simulink model "model_affc"  (R2016b)
settings: Solver=FixedStepDiscrete  StartTime=0.0  StopTime=inf  FixedStep=sampleTime  RelTol=1e-3
InitFcn:
  | model_affc_parameters;
StartFcn:
  | model_affc_parameters;
values from neighbouring files (symbols this model uses):
  Lb = 0.07    [model_affc_parameters.m]    (also in parameters_sysid.m)
  Lf = 0.238    [model_affc_parameters.m]    (also in parameters_sysid.m)
  Lu = 0.153    [model_affc_parameters.m]    (also in parameters_sysid.m)
  sampleTime = 0.001    [model_affc_parameters.m]    (also in parameters_sysid.m)
undefined symbols (not defined in the file or in its folder): FM1
libraries: simulink x4, LibraryFM x4, VariousBlocksLibrary x2, FMLibrary_v2 x1
settings Model: SimulationMode=external  Creator=niekbeckers  LastModifiedBy=Labuser
settings DataIOCC: LimitDataPoints=on  SaveFormat=Array
settings OptimizationCC: BlockReduction=off  BooleanDataType=off  LocalBlockOutputs=off  LifeSpan=inf
settings DebuggingCC: SaveWithParameterizedLinksMsg=none  UnderspecifiedInitializationDetection=Classic  MergeDetectMultiDrivingBlocksExec=none  SignalResolutionControl=TryResolveAllWithWarning  SFUnexpectedBacktrackingDiag=warning  SFNoUnconditionalDefaultTransitionDiag=warning  SFExecutionAtInitializationDiag=none
settings HardwareCC: ProdBitPerPointer=32  ProdBitPerSizeT=32  ProdBitPerPtrDiffT=32  ProdLargestAtomicFloat=None  ProdIntDivRoundTo=Undefined  ProdEndianess=Unspecified  ProdWordSize=32  ProdHWDeviceType=32-bit Generic  TargetBitPerPointer=64  TargetBitPerSizeT=64  TargetBitPerPtrDiffT=64  TargetLongLongMode=on  TargetIntDivRoundTo=Zero  TargetEndianess=LittleEndian  TargetWordSize=64  TargetHWDeviceType=MATLAB Host  ProdEqTarget=off
settings ModelReferenceCC: PropagateSignalLabelsOutOfModel=off
settings RTWCC: SystemTargetFile=TwinCAT.tlc  GenCodeOnly=on  MakeCommand=make_tct  TemplateMakefile=tct_msbuild.tmf  Description=TwinCAT Target  GenerateReport=on  TargetLang=C++
settings STFCustomTargetCC: CompOptLevelCompliant=on  GeneratePreprocessorConditionals=Disable all  MATLABClassNameForMDSCustomization=Simulink.SoftwareTarget.TargetSpecificTriggerConfigurationBase  SystemTargetFile=TwinCAT.tlc
settings ConfigComp: CovMetricSettings=dw  CovHtmlReporting=on  CovSaveCumulativeToWorkspaceVar=on  CovSaveSingleToWorkspaceVar=on  CovExternalEMLEnable=off  CovSFcnEnable=off

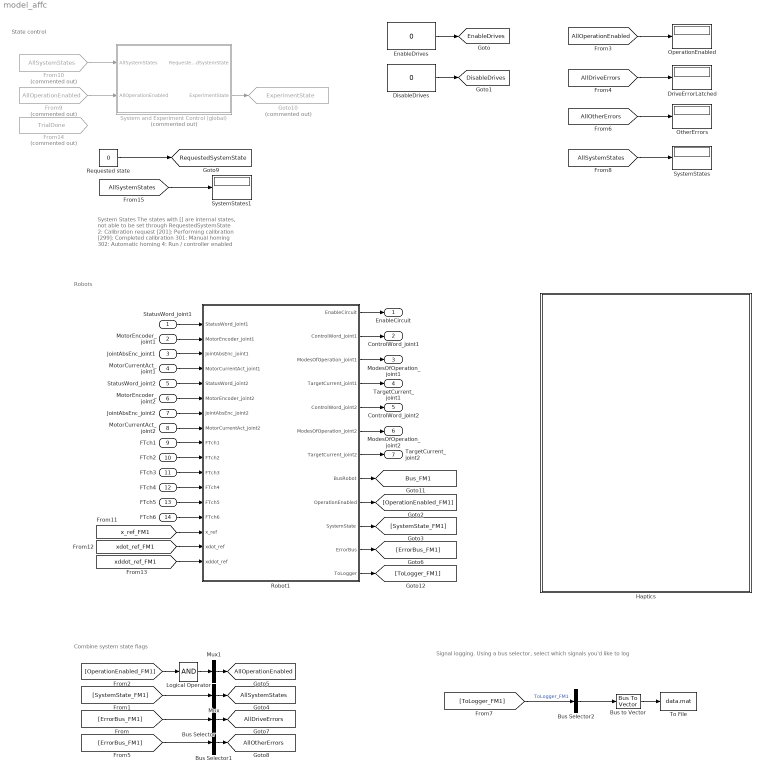
== system model_affc ==
  note: Signal logging.
      | Using a bus selector, select which signals you'd like to log
  note: System States
      | The states with [] are internal states, not able to be set through RequestedSystemState
      | 2: Calibration request
      | [201]: Performing calibration
      | [299]: Completed calibration
      | 301: Manual homing
      | 302: Automatic homing
      | 4: Run / controller enabled
  note: State control
  note: Combine system state flags
  note: Robots
  StatusWord_joint1 : Inport  OutDataTypeStr=uint16  PortDimensions=1
  MotorEncoder_joint1 : Inport  Port=2  OutDataTypeStr=int32  PortDimensions=1
  JointAbsEnc_joint1 : Inport  Port=3  OutDataTypeStr=int32  PortDimensions=1
  MotorCurrentAct_joint1 : Inport  Port=4  OutDataTypeStr=int16  PortDimensions=1
  StatusWord_joint2 : Inport  Port=5  OutDataTypeStr=uint16  PortDimensions=1
  MotorEncoder_joint2 : Inport  Port=6  OutDataTypeStr=int32  PortDimensions=1
  JointAbsEnc_joint2 : Inport  Port=7  OutDataTypeStr=int32  PortDimensions=1
  MotorCurrentAct_joint2 : Inport  Port=8  OutDataTypeStr=int16  PortDimensions=1
  FTch1 : Inport  Port=9  OutDataTypeStr=single  PortDimensions=1
  FTch2 : Inport  Port=10  OutDataTypeStr=single  PortDimensions=1
  FTch3 : Inport  Port=11  OutDataTypeStr=single  PortDimensions=1
  FTch4 : Inport  Port=12  OutDataTypeStr=single  PortDimensions=1
  FTch5 : Inport  Port=13  OutDataTypeStr=single  PortDimensions=1
  FTch6 : Inport  Port=14  OutDataTypeStr=single  PortDimensions=1
  Bus Selector : BusSelector  OutputSignals=DriveErrorLatched  OutputAsBus=on
  Bus Selector1 : BusSelector  OutputSignals=WorkspaceErrorLatched,ForceSensorLatched  OutputAsBus=on
  Bus Selector2 : BusSelector  OutputSignals=SystemState,ToLogger_ToEtherCAT.ToLogger_Actuator1.JointPosition_rad,ToLogger_ToEtherCAT.ToLogger_Actuator1.JointVelocity_rads,ToLogger_ToEtherCAT.ToLogger_Actuator1.JointTorque_Act_Nm,ToLogger_ToEtherCAT.ToLogger_Actuator1.DesiredTorqueLimited_Nm,ToLogger_ToEtherCAT.ToLogger_Actuator1.DriveError,ToLogger_ToEtherCAT.ToLogger_Actuator2.JointPosition_rad,ToLogger_ToEtherCAT.ToLogger_Actuator2.JointVelocity_rads,ToLogger_ToEtherCAT.ToLogger_Actuator2.JointTorque_Act_Nm,ToLogger_ToEtherCAT.ToLogger_Actuator2.DesiredTorqueLimited_Nm,ToLogger_ToEtherCAT.ToLogger_Actuator2.DriveError,ToLogger_Controller.q_ref,ToLogger_Controller.qdot_ref,ToLogger_Controller.qddot_ref  OutputAsBus=on
  Bus to Vector : BusToVector
  DisableDrives : Constant  Value=0
      settings: OpenFcn=set_param(gcb,'Value','1');tname = ['toggletimer_' gcb];delete(timerfind('name',tname));t = timer('timerfcn', ['set_param(''',gcb,''',''Value'',''0'')'],'executionmode','singleshot','startdelay',1,'name',tname);start(t);
      mask Display: fprintf('PushToTrigger\n%s',get_param(gcb,'value'))
  DriveErrorLatched : Display
  EnableDrives : Constant  Value=0
      settings: OpenFcn=set_param(gcb,'Value','1');tname = ['toggletimer_' gcb];delete(timerfind('name',tname));t = timer('timerfcn', ['set_param(''',gcb,''',''Value'',''0'')'],'executionmode','singleshot','startdelay',1,'name',tname);start(t);
      mask Display: fprintf('PushToTrigger\n%s',get_param(gcb,'value'))
  From10 : From  Commented=on  GotoTag=AllSystemStates
  From14 : From  Commented=on  GotoTag=TrialDone
  From9 : From  Commented=on  GotoTag=AllOperationEnabled
  Goto10 : Goto  Commented=on  GotoTag=ExperimentState  TagVisibility=global
  Haptics : Subsystem
  Logical Operator : Logic  Inputs=1  AllPortsSameDT=off  OutDataTypeStr=boolean
  Mux : Mux  Inputs=1
  Mux1 : Mux  Inputs=1
  OperationEnabled : Display
  OtherErrors : Display
  Requested state : Constant  Value=0
  Robot1 : Subsystem  AncestorBlock=LibraryFM/Robot1  mask{RobotStruct=FM1}
      mask prompts: RobotStruct "Robot struct (data)"
  System and Experiment Control (global) : Subsystem  Commented=on
  SystemStates : Display
  SystemStates1 : Display
  To File : ToFile  Filename=data.mat
  EnableCircuit : Outport  OutDataTypeStr=boolean  PortDimensions=1
  ControlWord_joint1 : Outport  Port=2  OutDataTypeStr=uint16  PortDimensions=1
  ModesOfOperation_joint1 : Outport  Port=3  OutDataTypeStr=int8  PortDimensions=1
  TargetCurrent_joint1 : Outport  Port=4  OutDataTypeStr=int16  PortDimensions=1
  ControlWord_joint2 : Outport  Port=5  OutDataTypeStr=uint16  PortDimensions=1
  ModesOfOperation_joint2 : Outport  Port=6  OutDataTypeStr=int8  PortDimensions=1
  TargetCurrent_joint2 : Outport  Port=7  OutDataTypeStr=int16  PortDimensions=1
  tag scope: AllDriveErrors=global, AllOperationEnabled=global, AllOtherErrors=global, AllSystemStates=global, Bus_FM1=global, DisableDrives=global, EnableDrives=global, RequestedSystemState=global
  wires:
  DisableDrives/1 -> [DisableDrives]
  EnableDrives/1 -> [EnableDrives]
  Robot1/9(OperationEnabled) -> [OperationEnabled_FM1]
  [AllOperationEnabled] -> OperationEnabled/1
  Robot1/10(SystemState) -> [SystemState_FM1]
  [SystemState_FM1] -> Mux/1
  Mux/1 -> [AllSystemStates]
  Mux1/1 -> [AllOperationEnabled]
  [OperationEnabled_FM1] -> Logical Operator/1
  Robot1/11(ErrorBus) -> [ErrorBus_FM1]
  [ErrorBus_FM1] -> Bus Selector/1
  Bus Selector/1 -> [AllDriveErrors]
  [AllDriveErrors] -> DriveErrorLatched/1
  [ErrorBus_FM1] -> Bus Selector1/1
  Bus Selector1/1 -> [AllOtherErrors]
  [AllOtherErrors] -> OtherErrors/1
  [AllSystemStates] -> SystemStates/1
  System and Experiment Control (global)/2(ExperimentState) -> Goto10/1
  From10/1 -> System and Experiment Control (global)/1(AllSystemStates)
  From9/1 -> System and Experiment Control (global)/2(AllOperationEnabled)
  [x_ref_FM1] -> Robot1/15(x_ref)
  [xdot_ref_FM1] -> Robot1/16(xdot_ref)
  [xddot_ref_FM1] -> Robot1/17(xddot_ref)
  Requested state/1 -> [RequestedSystemState]
  Robot1/8(BusRobot) -> [Bus_FM1]
  StatusWord_joint1/1 -> Robot1/1(StatusWord_joint1)
  MotorEncoder_joint1/1 -> Robot1/2(MotorEncoder_joint1)
  JointAbsEnc_joint1/1 -> Robot1/3(JointAbsEnc_joint1)
  MotorCurrentAct_joint1/1 -> Robot1/4(MotorCurrentAct_joint1)
  StatusWord_joint2/1 -> Robot1/5(StatusWord_joint2)
  MotorEncoder_joint2/1 -> Robot1/6(MotorEncoder_joint2)
  JointAbsEnc_joint2/1 -> Robot1/7(JointAbsEnc_joint2)
  MotorCurrentAct_joint2/1 -> Robot1/8(MotorCurrentAct_joint2)
  FTch1/1 -> Robot1/9(FTch1)
  FTch2/1 -> Robot1/10(FTch2)
  FTch3/1 -> Robot1/11(FTch3)
  FTch4/1 -> Robot1/12(FTch4)
  FTch5/1 -> Robot1/13(FTch5)
  FTch6/1 -> Robot1/14(FTch6)
  Robot1/1(EnableCircuit) -> EnableCircuit/1
  Robot1/2(ControlWord_joint1) -> ControlWord_joint1/1
  Robot1/3(ModesOfOperation_joint1) -> ModesOfOperation_joint1/1
  Robot1/4(TargetCurrent_joint1) -> TargetCurrent_joint1/1
  Robot1/7(TargetCurrent_joint2) -> TargetCurrent_joint2/1
  Robot1/6(ModesOfOperation_joint2) -> ModesOfOperation_joint2/1
  Robot1/5(ControlWord_joint2) -> ControlWord_joint2/1
  Robot1/12(ToLogger) -> [ToLogger_FM1]
  [ToLogger_FM1] -> Bus Selector2/1  "ToLogger_FM1"
  Bus Selector2/1 -> Bus to Vector/1
  Bus to Vector/1 -> To File/1
  Logical Operator/1 -> Mux1/1
  [AllSystemStates] -> SystemStates1/1

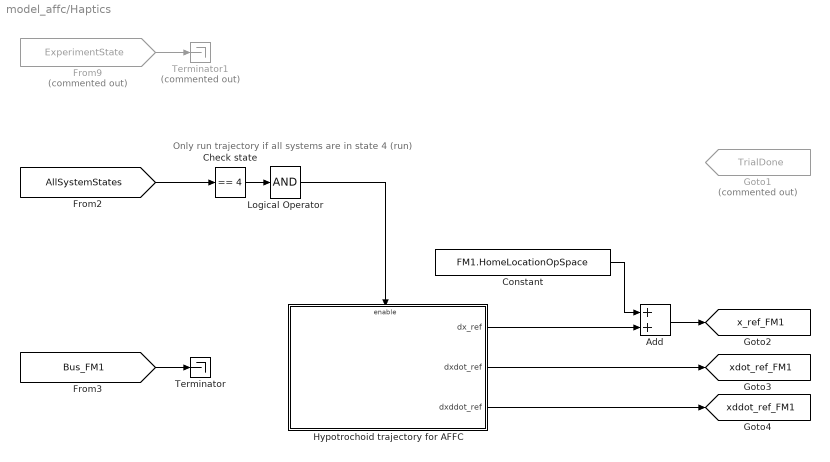
== system model_affc/Haptics ==
  note: Only run trajectory if all systems are in state 4 (run)
  Add : Sum
  "Check state " : simulink/Logic and Bit Operations/Compare To Constant  relop===  const=4  OutDataTypeStr=boolean
  Constant : Constant  Value=FM1.HomeLocationOpSpace
  From9 : From  Commented=on  GotoTag=ExperimentState
  Goto1 : Goto  Commented=on  GotoTag=TrialDone  TagVisibility=global
  Hypotrochoid trajectory for AFFC : Subsystem
  Logical Operator : Logic  Inputs=1  AllPortsSameDT=off  OutDataTypeStr=boolean
  Terminator : Terminator
  Terminator1 : Terminator  Commented=on
  tag scope: x_ref_FM1=global, xddot_ref_FM1=global, xdot_ref_FM1=global
  wires:
  [Bus_FM1] -> Terminator/1
  Constant/1 -> Add/1
  Hypotrochoid trajectory for AFFC/1(dx_ref) -> Add/2
  Add/1 -> [x_ref_FM1]
  Hypotrochoid trajectory for AFFC/2(dxdot_ref) -> [xdot_ref_FM1]
  Hypotrochoid trajectory for AFFC/3(dxddot_ref) -> [xddot_ref_FM1]
  [AllSystemStates] -> "Check state "/1
  "Check state "/1 -> Logical Operator/1
  Logical Operator/1 -> Hypotrochoid trajectory for AFFC/Enable
  From9/1 -> Terminator1/1

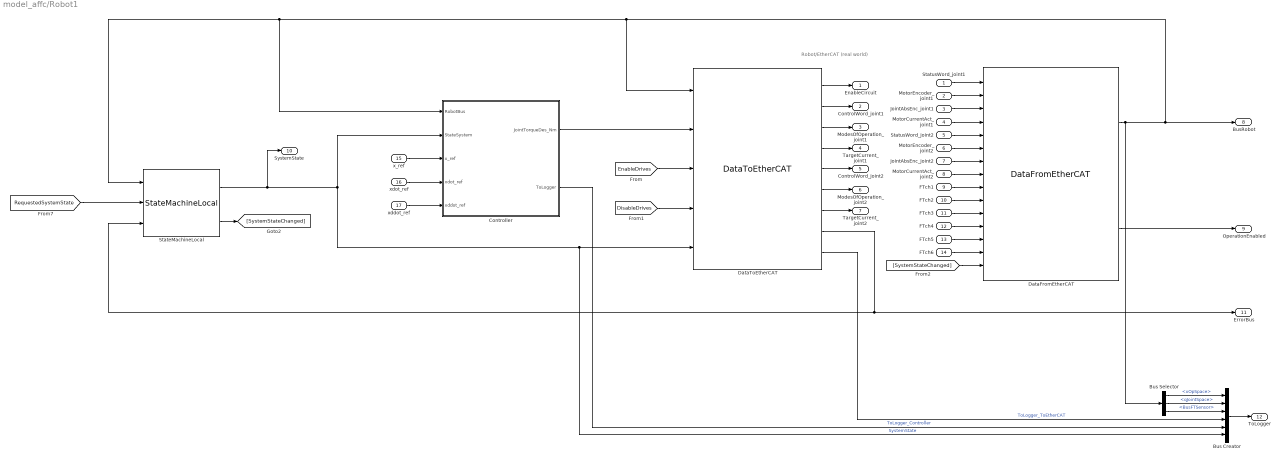
== system model_affc/Robot1 ==
  note: Robot/EtherCAT (real world)
  StatusWord_joint1 : Inport
  MotorEncoder_joint1 : Inport  Port=2
  JointAbsEnc_joint1 : Inport  Port=3
  MotorCurrentAct_joint1 : Inport  Port=4
  StatusWord_joint2 : Inport  Port=5
  MotorEncoder_joint2 : Inport  Port=6
  JointAbsEnc_joint2 : Inport  Port=7
  MotorCurrentAct_joint2 : Inport  Port=8
  FTch1 : Inport  Port=9
  FTch2 : Inport  Port=10
  FTch3 : Inport  Port=11
  FTch4 : Inport  Port=12
  FTch5 : Inport  Port=13
  FTch6 : Inport  Port=14
  x_ref : Inport  Port=15
  xdot_ref : Inport  Port=16
  xddot_ref : Inport  Port=17
  Bus Creator : BusCreator  Inputs=6
  Bus Selector : BusSelector  OutputSignals=xOpSpace,qJointSpace,BusFTSensor
  Controller : Subsystem  AncestorBlock=LibraryFM/Controller
  DataFromEtherCAT : LibraryFM/DataFromEtherCAT
  DataToEtherCAT : LibraryFM/DataToEtherCAT
  StateMachineLocal : LibraryFM/StateMachineLocal
  EnableCircuit : Outport
  ControlWord_joint1 : Outport  Port=2
  ModesOfOperation_joint1 : Outport  Port=3
  TargetCurrent_joint1 : Outport  Port=4
  ControlWord_joint2 : Outport  Port=5
  ModesOfOperation_joint2 : Outport  Port=6
  TargetCurrent_joint2 : Outport  Port=7
  BusRobot : Outport  Port=8
  OperationEnabled : Outport  Port=9
  SystemState : Outport  Port=10
  ErrorBus : Outport  Port=11
  ToLogger : Outport  Port=12
  wires:
  Controller/2(ToLogger) -> Bus Creator/5  "ToLogger_Controller"
  DataToEtherCAT/9 -> Bus Creator/4  "ToLogger_ToEtherCAT"
  Bus Creator/1 -> ToLogger/1
  xddot_ref/1 -> Controller/5(xddot_ref)
  xdot_ref/1 -> Controller/4(xdot_ref)
  x_ref/1 -> Controller/3(x_ref)
  DataToEtherCAT/7 -> TargetCurrent_joint2/1
  FTch2/1 -> DataFromEtherCAT/10
  MotorCurrentAct_joint1/1 -> DataFromEtherCAT/4
  MotorEncoder_joint2/1 -> DataFromEtherCAT/6
  JointAbsEnc_joint1/1 -> DataFromEtherCAT/3
  DataToEtherCAT/3 -> ModesOfOperation_joint1/1
  DataToEtherCAT/1 -> EnableCircuit/1
  FTch1/1 -> DataFromEtherCAT/9
  StateMachineLocal/1 -> Bus Creator/6, DataToEtherCAT/5, Controller/2(StateSystem), SystemState/1  "SystemState"
  DataToEtherCAT/2 -> ControlWord_joint1/1
  StateMachineLocal/2 -> [SystemStateChanged]
  [SystemStateChanged] -> DataFromEtherCAT/15
  DataToEtherCAT/8 -> ErrorBus/1, StateMachineLocal/3
  DataFromEtherCAT/1 -> Bus Selector/1, StateMachineLocal/1, Controller/1(RobotBus), DataToEtherCAT/1, BusRobot/1
  [RequestedSystemState] -> StateMachineLocal/2
  Controller/1(JointTorqueDes_Nm) -> DataToEtherCAT/2
  [DisableDrives] -> DataToEtherCAT/4
  [EnableDrives] -> DataToEtherCAT/3
  MotorCurrentAct_joint2/1 -> DataFromEtherCAT/8
  DataToEtherCAT/4 -> TargetCurrent_joint1/1
  FTch5/1 -> DataFromEtherCAT/13
  JointAbsEnc_joint2/1 -> DataFromEtherCAT/7
  MotorEncoder_joint1/1 -> DataFromEtherCAT/2
  DataToEtherCAT/5 -> ControlWord_joint2/1
  DataToEtherCAT/6 -> ModesOfOperation_joint2/1
  StatusWord_joint1/1 -> DataFromEtherCAT/1
  StatusWord_joint2/1 -> DataFromEtherCAT/5
  FTch6/1 -> DataFromEtherCAT/14
  FTch4/1 -> DataFromEtherCAT/12
  FTch3/1 -> DataFromEtherCAT/11
  DataFromEtherCAT/2 -> OperationEnabled/1
  Bus Selector/3 -> Bus Creator/3  "<BusFTSensor>"
  Bus Selector/2 -> Bus Creator/2  "<qJointSpace>"
  Bus Selector/1 -> Bus Creator/1  "<xOpSpace>"

== system model_affc/System and Experiment Control (global) ==
  note: Hier ergens experiment protocol inlezen
  AllSystemStates : Inport
  AllOperationEnabled : Inport  Port=2
  GlobalStateMachine : FMLibrary_v2/StateMachineLocal/SystemLocalStateMachine
  RequestedSystemState : Outport
  ExperimentState : Outport  Port=2
  wires:
  GlobalStateMachine/1 -> RequestedSystemState/1

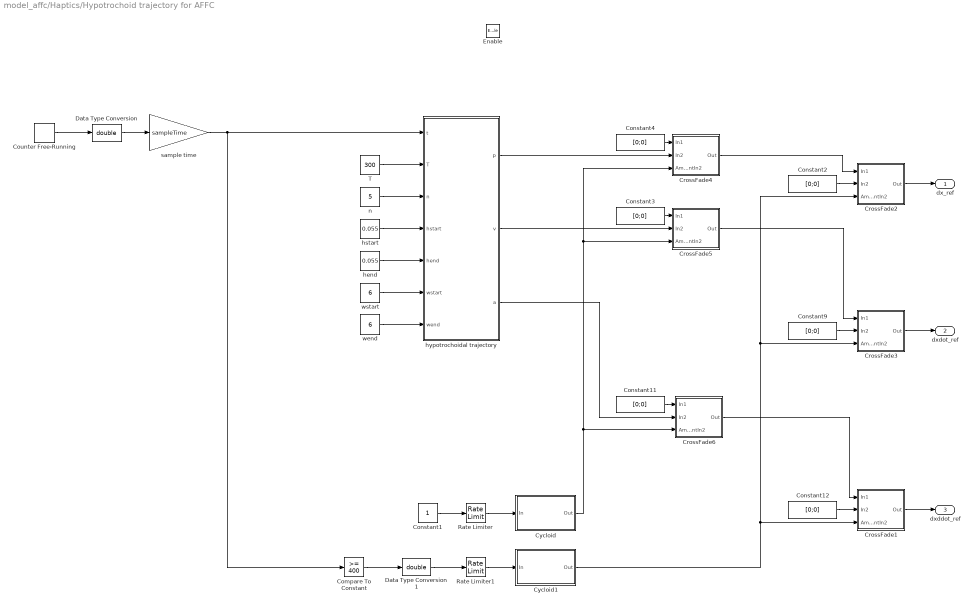
== system model_affc/Haptics/Hypotrochoid trajectory for AFFC ==
  Enable : EnablePort  StatesWhenEnabling=reset
  Compare To Constant : simulink/Logic and Bit Operations/Compare To Constant  relop=>=  const=400  OutDataTypeStr=boolean
  Constant1 : Constant
  Constant{2..4,9,11..12} (6 alike) : Constant  Value=[0;0]
  Counter Free-Running : simulink/Sources/Counter Free-Running  NumBits=32  tsamp=-1
  CrossFade1 : Subsystem  AncestorBlock=VariousBlocksLibrary/Various/CrossFade
  CrossFade2 : Subsystem  AncestorBlock=VariousBlocksLibrary/Various/CrossFade
  CrossFade3 : Subsystem  AncestorBlock=VariousBlocksLibrary/Various/CrossFade
  CrossFade4 : Subsystem
  CrossFade5 : Subsystem  AncestorBlock=VariousBlocksLibrary/Various/CrossFade
  CrossFade6 : Subsystem  AncestorBlock=VariousBlocksLibrary/Various/CrossFade
  Cycloid : Subsystem  AncestorBlock=VariousBlocksLibrary/Various/Cycloid
  Cycloid1 : Subsystem  AncestorBlock=VariousBlocksLibrary/Various/Cycloid
  Data Type Conversion : DataTypeConversion  OutDataTypeStr=double
  Data Type Conversion1 : DataTypeConversion  OutDataTypeStr=double
  Rate Limiter : RateLimiter  RisingSlewLimit=0.25  FallingSlewLimit=-0.15  SampleTimeMode=inherited
  Rate Limiter1 : RateLimiter  RisingSlewLimit=0.2  FallingSlewLimit=-0.2  SampleTimeMode=inherited
  T : Constant  Value=300
  hend : Constant  Value=0.055
  hstart : Constant  Value=0.055
  hypotrochoidal trajectory : MATLAB Function  TreatAsAtomicUnit=on
  n : Constant  Value=5
  sample time : Gain  Gain=sampleTime
  wend : Constant  Value=6
  wstart : Constant  Value=6
  dx_ref : Outport
  dxdot_ref : Outport  Port=2
  dxddot_ref : Outport  Port=3
  wires:
  Data Type Conversion1/1 -> Rate Limiter1/1
  hypotrochoidal trajectory/1(p) -> CrossFade4/2(In2)
  CrossFade1/1(Out) -> dxddot_ref/1
  Constant11/1 -> CrossFade6/1(In1)
  Constant12/1 -> CrossFade1/2(In2)
  CrossFade6/1(Out) -> CrossFade1/1(In1)
  Constant9/1 -> CrossFade3/2(In2)
  CrossFade5/1(Out) -> CrossFade3/1(In1)
  CrossFade3/1(Out) -> dxdot_ref/1
  Cycloid1/1(Out) -> CrossFade1/3(AmountIn2), CrossFade2/3(AmountIn2), CrossFade3/3(AmountIn2)
  Rate Limiter1/1 -> Cycloid1/1(In)
  Compare To Constant/1 -> Data Type Conversion1/1
  CrossFade4/1(Out) -> CrossFade2/1(In1)
  CrossFade2/1(Out) -> dx_ref/1
  Rate Limiter/1 -> Cycloid/1(In)
  Constant1/1 -> Rate Limiter/1
  Cycloid/1(Out) -> CrossFade6/3(AmountIn2), CrossFade5/3(AmountIn2), CrossFade4/3(AmountIn2)
  hypotrochoidal trajectory/2(v) -> CrossFade5/2(In2)
  hypotrochoidal trajectory/3(a) -> CrossFade6/2(In2)
  sample time/1 -> Compare To Constant/1, hypotrochoidal trajectory/1(t)
  Constant2/1 -> CrossFade2/2(In2)
  Data Type Conversion/1 -> sample time/1
  wstart/1 -> hypotrochoidal trajectory/6(wstart)
  wend/1 -> hypotrochoidal trajectory/7(wend)
  hstart/1 -> hypotrochoidal trajectory/4(hstart)
  hend/1 -> hypotrochoidal trajectory/5(hend)
  n/1 -> hypotrochoidal trajectory/3(n)
  T/1 -> hypotrochoidal trajectory/2(T)
  Counter Free-Running/1 -> Data Type Conversion/1
  Constant3/1 -> CrossFade5/1(In1)
  Constant4/1 -> CrossFade4/1(In1)

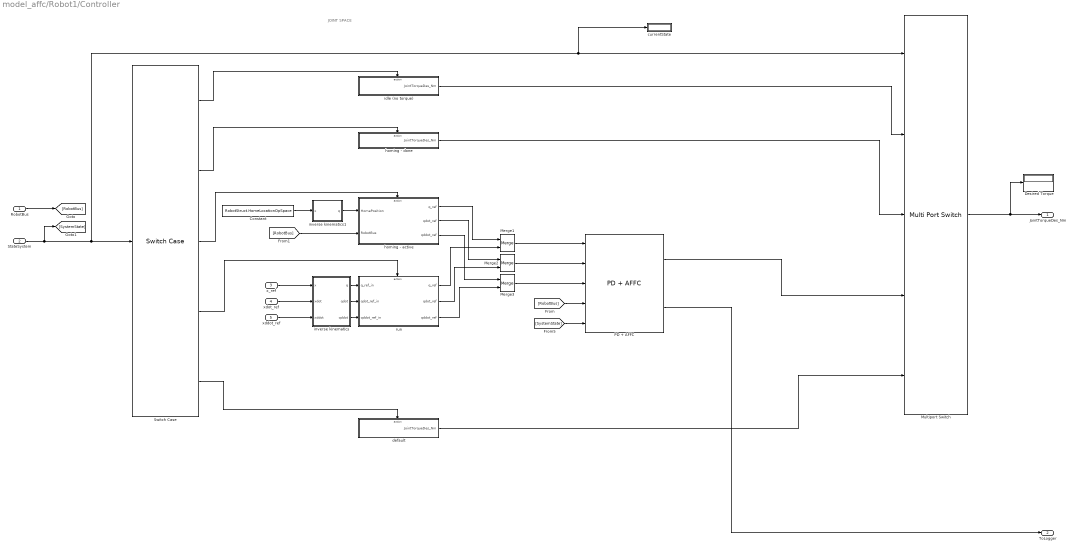
== system model_affc/Robot1/Controller ==
  note: JOINT SPACE
  RobotBus : Inport
  StateSystem : Inport  Port=2
  x_ref : Inport  Port=3
  xdot_ref : Inport  Port=4
  xddot_ref : Inport  Port=5
  Constant : Constant  Value=RobotStruct.HomeLocationOpSpace
  Desired Torque : Display
  Merge1 : Merge
  Merge2 : Merge
  Merge3 : Merge
  Multiport Switch : MultiPortSwitch  DataPortOrder=Specify indices  Inputs=4  DataPortIndices={[0,1,2,201,299,301],[399],[302,4]}  DataPortForDefault=Additional data port
  PD + AFFC : LibraryFM/PD + AFFC
      link override AFFC/p: InitialOutput=zeros(7,1)
  Switch Case : SwitchCase  CaseConditions={[0,1,2,201,299,301],[399],[302],[4]}
  currentState : Display
  default : Subsystem  TreatAsAtomicUnit=on
  homing - active : Subsystem
  homing - done : Subsystem  TreatAsAtomicUnit=on
  idle (no torque) : Subsystem  TreatAsAtomicUnit=on
  inverse kinematics : MATLAB Function  TreatAsAtomicUnit=on
  inverse kinematics1 : MATLAB Function  TreatAsAtomicUnit=on
  run : Subsystem
  JointTorqueDes_Nm : Outport
  ToLogger : Outport  Port=2
  wires:
  PD + AFFC/2 -> ToLogger/1
  xdot_ref/1 -> inverse kinematics/2(xdot)
  xddot_ref/1 -> inverse kinematics/3(xddot)
  x_ref/1 -> inverse kinematics/1(x)
  [SystemState] -> PD + AFFC/5
  inverse kinematics1/1(q) -> homing - active/1(HomePosition)
  inverse kinematics/3(qddot) -> run/3(qddot_ref_in)
  inverse kinematics/2(qdot) -> run/2(qdot_ref_in)
  inverse kinematics/1(q) -> run/1(q_ref_in)
  Constant/1 -> inverse kinematics1/1(x)
  [RobotBus] -> homing - active/2(RobotBus)
  [RobotBus] -> PD + AFFC/4
  RobotBus/1 -> [RobotBus]
  PD + AFFC/1 -> Multiport Switch/4
  Merge3/1 -> PD + AFFC/3
  Merge2/1 -> PD + AFFC/2
  Merge1/1 -> PD + AFFC/1
  homing - done/1(JointTorqueDes_Nm) -> Multiport Switch/3
  idle (no torque)/1(JointTorqueDes_Nm) -> Multiport Switch/2
  Switch Case/2 -> homing - done/Action
  Switch Case/3 -> homing - active/Action
  Switch Case/1 -> idle (no torque)/Action
  default/1(JointTorqueDes_Nm) -> Multiport Switch/5
  Switch Case/5 -> default/Action
  Multiport Switch/1 -> Desired Torque/1, JointTorqueDes_Nm/1
  Switch Case/4 -> run/Action
  homing - active/1(q_ref) -> Merge1/1
  run/1(q_ref) -> Merge1/2
  StateSystem/1 -> Multiport Switch/1, currentState/1, Switch Case/1, [SystemState]
  run/2(qdot_ref) -> Merge2/2
  run/3(qddot_ref) -> Merge3/2
  homing - active/2(qdot_ref) -> Merge2/1
  homing - active/3(qddot_ref) -> Merge3/1

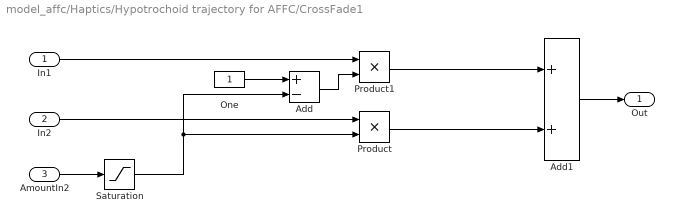
== system model_affc/Haptics/Hypotrochoid trajectory for AFFC/CrossFade1 ==
  In1 : Inport
  In2 : Inport  Port=2
  AmountIn2 : Inport  Port=3
  Add : Sum  Inputs=+-
  Add1 : Sum
  One : Constant
  Product : Product  RndMeth=Zero
  Product1 : Product  RndMeth=Zero
  Saturation : Saturate  UpperLimit=1  LowerLimit=0
  Out : Outport
  wires:
  In1/1 -> Product1/1
  AmountIn2/1 -> Saturation/1
  One/1 -> Add/1
  Saturation/1 -> Product/2, Add/2
  Add/1 -> Product1/2
  Product/1 -> Add1/2
  Product1/1 -> Add1/1
  In2/1 -> Product/1
  Add1/1 -> Out/1

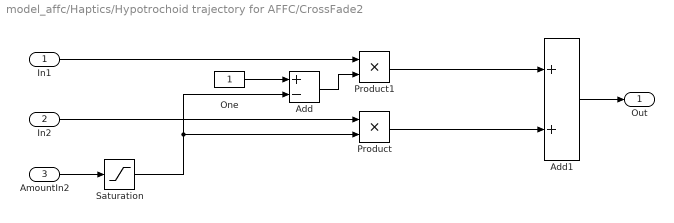
== system model_affc/Haptics/Hypotrochoid trajectory for AFFC/CrossFade2 ==
  In1 : Inport
  In2 : Inport  Port=2
  AmountIn2 : Inport  Port=3
  Add : Sum  Inputs=+-
  Add1 : Sum
  One : Constant
  Product : Product  RndMeth=Zero
  Product1 : Product  RndMeth=Zero
  Saturation : Saturate  UpperLimit=1  LowerLimit=0
  Out : Outport
  wires:
  In1/1 -> Product1/1
  AmountIn2/1 -> Saturation/1
  One/1 -> Add/1
  Saturation/1 -> Product/2, Add/2
  Add/1 -> Product1/2
  Product/1 -> Add1/2
  Product1/1 -> Add1/1
  In2/1 -> Product/1
  Add1/1 -> Out/1

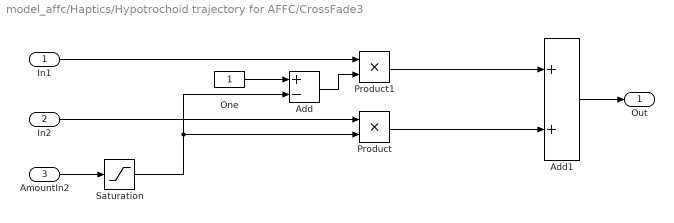
== system model_affc/Haptics/Hypotrochoid trajectory for AFFC/CrossFade3 ==
  In1 : Inport
  In2 : Inport  Port=2
  AmountIn2 : Inport  Port=3
  Add : Sum  Inputs=+-
  Add1 : Sum
  One : Constant
  Product : Product  RndMeth=Zero
  Product1 : Product  RndMeth=Zero
  Saturation : Saturate  UpperLimit=1  LowerLimit=0
  Out : Outport
  wires:
  In1/1 -> Product1/1
  AmountIn2/1 -> Saturation/1
  One/1 -> Add/1
  Saturation/1 -> Product/2, Add/2
  Add/1 -> Product1/2
  Product/1 -> Add1/2
  Product1/1 -> Add1/1
  In2/1 -> Product/1
  Add1/1 -> Out/1

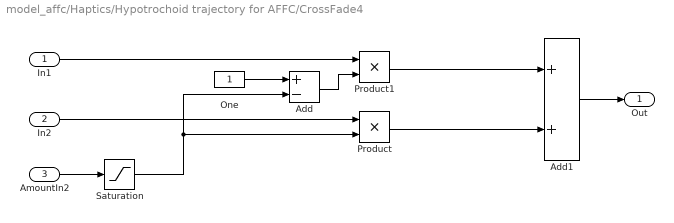
== system model_affc/Haptics/Hypotrochoid trajectory for AFFC/CrossFade4 ==
  In1 : Inport
  In2 : Inport  Port=2
  AmountIn2 : Inport  Port=3
  Add : Sum  Inputs=+-
  Add1 : Sum
  One : Constant
  Product : Product  RndMeth=Zero
  Product1 : Product  RndMeth=Zero
  Saturation : Saturate  UpperLimit=1  LowerLimit=0
  Out : Outport
  wires:
  In1/1 -> Product1/1
  AmountIn2/1 -> Saturation/1
  One/1 -> Add/1
  Saturation/1 -> Product/2, Add/2
  Add/1 -> Product1/2
  Product/1 -> Add1/2
  Product1/1 -> Add1/1
  In2/1 -> Product/1
  Add1/1 -> Out/1

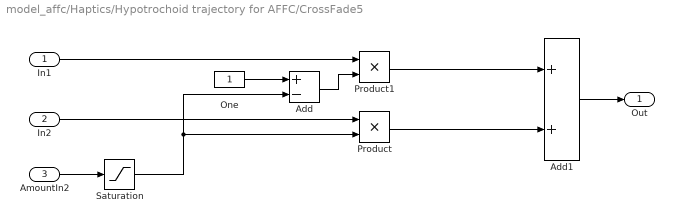
== system model_affc/Haptics/Hypotrochoid trajectory for AFFC/CrossFade5 ==
  In1 : Inport
  In2 : Inport  Port=2
  AmountIn2 : Inport  Port=3
  Add : Sum  Inputs=+-
  Add1 : Sum
  One : Constant
  Product : Product  RndMeth=Zero
  Product1 : Product  RndMeth=Zero
  Saturation : Saturate  UpperLimit=1  LowerLimit=0
  Out : Outport
  wires:
  In1/1 -> Product1/1
  AmountIn2/1 -> Saturation/1
  One/1 -> Add/1
  Saturation/1 -> Product/2, Add/2
  Add/1 -> Product1/2
  Product/1 -> Add1/2
  Product1/1 -> Add1/1
  In2/1 -> Product/1
  Add1/1 -> Out/1

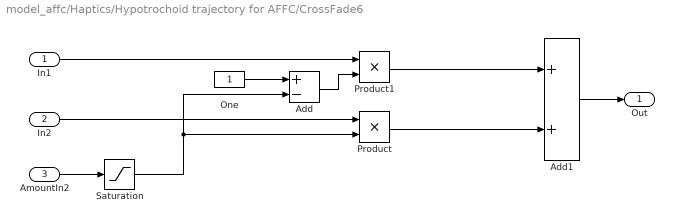
== system model_affc/Haptics/Hypotrochoid trajectory for AFFC/CrossFade6 ==
  In1 : Inport
  In2 : Inport  Port=2
  AmountIn2 : Inport  Port=3
  Add : Sum  Inputs=+-
  Add1 : Sum
  One : Constant
  Product : Product  RndMeth=Zero
  Product1 : Product  RndMeth=Zero
  Saturation : Saturate  UpperLimit=1  LowerLimit=0
  Out : Outport
  wires:
  In1/1 -> Product1/1
  AmountIn2/1 -> Saturation/1
  One/1 -> Add/1
  Saturation/1 -> Product/2, Add/2
  Add/1 -> Product1/2
  Product/1 -> Add1/2
  Product1/1 -> Add1/1
  In2/1 -> Product/1
  Add1/1 -> Out/1

== system model_affc/Haptics/Hypotrochoid trajectory for AFFC/Cycloid ==
  note: Given a linear input 0<=in<=1, it gives a cycloid output 0<=out<=1.
      | If In is outside the 0..1 range, it is limited to 0 or 1.
  In : Inport
  Gain1 : Gain  Gain=2*pi
  Gain2 : Gain  Gain=1/(2*pi)
  Saturation : Saturate  UpperLimit=1  LowerLimit=0
  Subtract : Sum  Inputs=+-
  Trigonometric Function : Trigonometry
  Out : Outport
  wires:
  Gain1/1 -> Trigonometric Function/1
  Subtract/1 -> Out/1
  In/1 -> Saturation/1
  Saturation/1 -> Gain1/1, Subtract/1
  Trigonometric Function/1 -> Gain2/1
  Gain2/1 -> Subtract/2

== system model_affc/Haptics/Hypotrochoid trajectory for AFFC/Cycloid1 ==
  note: Given a linear input 0<=in<=1, it gives a cycloid output 0<=out<=1.
      | If In is outside the 0..1 range, it is limited to 0 or 1.
  In : Inport
  Gain1 : Gain  Gain=2*pi
  Gain2 : Gain  Gain=1/(2*pi)
  Saturation : Saturate  UpperLimit=1  LowerLimit=0
  Subtract : Sum  Inputs=+-
  Trigonometric Function : Trigonometry
  Out : Outport
  wires:
  Gain1/1 -> Trigonometric Function/1
  Subtract/1 -> Out/1
  In/1 -> Saturation/1
  Saturation/1 -> Gain1/1, Subtract/1
  Trigonometric Function/1 -> Gain2/1
  Gain2/1 -> Subtract/2

== system model_affc/Robot1/Controller/default ==
  Action Port : ActionPort  InitializeStates=reset  ActionType=default
  Constant3 : Constant  Value=[0;0]
  JointTorqueDes_Nm : Outport  InitialOutput=[0;0]
  wires:
  Constant3/1 -> JointTorqueDes_Nm/1

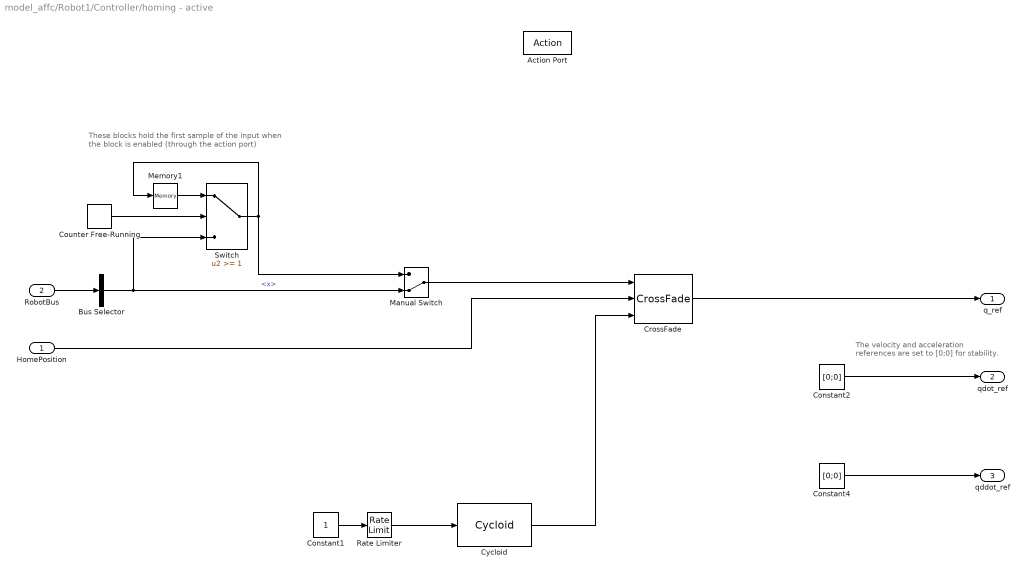
== system model_affc/Robot1/Controller/homing - active ==
  note: These blocks hold the first sample of the input
      | when the block is enabled (through the action port)
  note: The velocity and acceleration references are set to [0;0] for stability.
  HomePosition : Inport
  RobotBus : Inport  Port=2
  Action Port : ActionPort  InitializeStates=reset  ActionType=case
  Bus Selector : BusSelector  OutputSignals=xOpSpace.x
  Constant1 : Constant
  Constant2 : Constant  Value=[0;0]
  Constant4 : Constant  Value=[0;0]
  Counter Free-Running : simulink/Sources/Counter Free-Running  NumBits=32  tsamp=-1
  CrossFade : VariousBlocksLibrary/Various/CrossFade
  Cycloid : VariousBlocksLibrary/Various/Cycloid
  Manual Switch : ManualSwitch  CurrentSetting=0
  Memory1 : Memory
  Rate Limiter : RateLimiter  RisingSlewLimit=0.2  FallingSlewLimit=-0.2  SampleTimeMode=inherited
  Switch : Switch  Threshold=1
  q_ref : Outport  OutputWhenDisabled=reset  InitialOutput=[0;0]
  qdot_ref : Outport  Port=2  OutputWhenDisabled=reset  InitialOutput=[0;0]
  qddot_ref : Outport  Port=3  OutputWhenDisabled=reset  InitialOutput=[0;0]
  wires:
  Constant2/1 -> qdot_ref/1
  Bus Selector/1 -> Manual Switch/2, Switch/3  "<x>"
  RobotBus/1 -> Bus Selector/1
  HomePosition/1 -> CrossFade/2
  Cycloid/1 -> CrossFade/3
  Rate Limiter/1 -> Cycloid/1
  Constant1/1 -> Rate Limiter/1
  Switch/1 -> Memory1/1, Manual Switch/1
  Counter Free-Running/1 -> Switch/2
  Memory1/1 -> Switch/1
  Manual Switch/1 -> CrossFade/1
  CrossFade/1 -> q_ref/1
  Constant4/1 -> qddot_ref/1

== system model_affc/Robot1/Controller/homing - done ==
  Action Port : ActionPort  ActionType=case
  Constant : Constant  Value=[0;0]
  JointTorqueDes_Nm : Outport  InitialOutput=[0;0]
  wires:
  Constant/1 -> JointTorqueDes_Nm/1

== system model_affc/Robot1/Controller/idle (no torque) ==
  Action Port : ActionPort  InitializeStates=reset  ActionType=case
  Constant3 : Constant  Value=[0;0]
  JointTorqueDes_Nm : Outport  InitialOutput=[0;0]
  wires:
  Constant3/1 -> JointTorqueDes_Nm/1

== system model_affc/Robot1/Controller/run ==
  q_ref_in : Inport
  qdot_ref_in : Inport  Port=2
  qddot_ref_in : Inport  Port=3
  Action Port : ActionPort  InitializeStates=reset  ActionType=case
  q_ref : Outport  OutputWhenDisabled=reset  InitialOutput=[0;0]
  qdot_ref : Outport  Port=2  OutputWhenDisabled=reset  InitialOutput=[0;0]
  qddot_ref : Outport  Port=3  OutputWhenDisabled=reset  InitialOutput=[0;0]
  wires:
  qdot_ref_in/1 -> qdot_ref/1
  qddot_ref_in/1 -> qddot_ref/1
  q_ref_in/1 -> q_ref/1

== matlab function model_affc/Robot1/Controller/inverse kinematics1 ==
  data: x input; q output size=[2 1]; Lf parameter; Lu parameter; Lb parameter
function q  = IK(x,Lf,Lu,Lb)
%#codegen

% inverse dynamics
q = func_eq_IK(x(1),x(2),Lf,Lu,Lb);

== matlab function model_affc/Haptics/Hypotrochoid trajectory for AFFC/hypotrochoidal trajectory ==
  data: t input; p output; v output; a output; T input; n input; hstart input; hend input; wstart input; wend input
function [p,v,a] = fcn(t,T,n,hstart,hend,wstart,wend)
%#codegen

p = func_p_hypothrochoid(t,T,n,hstart,hend,wstart,wend);
v = func_v_hypothrochoid(t,T,n,hstart,hend,wstart,wend);
a = func_a_hypothrochoid(t,T,n,hstart,hend,wstart,wend);

== matlab function model_affc/Robot1/Controller/inverse kinematics ==
  data: x input; xdot input; xddot input; q output size=[2 1]; Lf parameter; Lu parameter; Lb parameter; qdot output; qddot output
function [q,qdot,qddot] = IK(x,xdot,xddot,Lf,Lu,Lb)
%#codegen

% inverse dynamics
q = func_eq_IK(x(1),x(2),Lf,Lu,Lb);

% jacobians
Je = func_eq_Je(q(1),q(2),Lf,Lu,Lb);

% calculate qdot
qdot = pinv(Je)*xdot;

% calculate qddot
Jedot = func_eq_Jedot(q(1),q(2),qdot(1),qdot(2),Lf,Lu,Lb);
qddot = pinv(Je)*(xddot-Jedot*qdot);
